simulink model "Motor_Position"  (R2020b)
settings: Solver=ode15s  StartTime=0.0  StopTime=0.2  RelTol=1e-3
undefined symbols (not defined in the file): b, J, Ke, Kt, L, R
settings Model: DataDictionary=motor_pos_data.sldd  Creator=ADMIN  LastModifiedBy=ADMIN
settings DataIOCC: SaveOutput=off  SaveTime=off

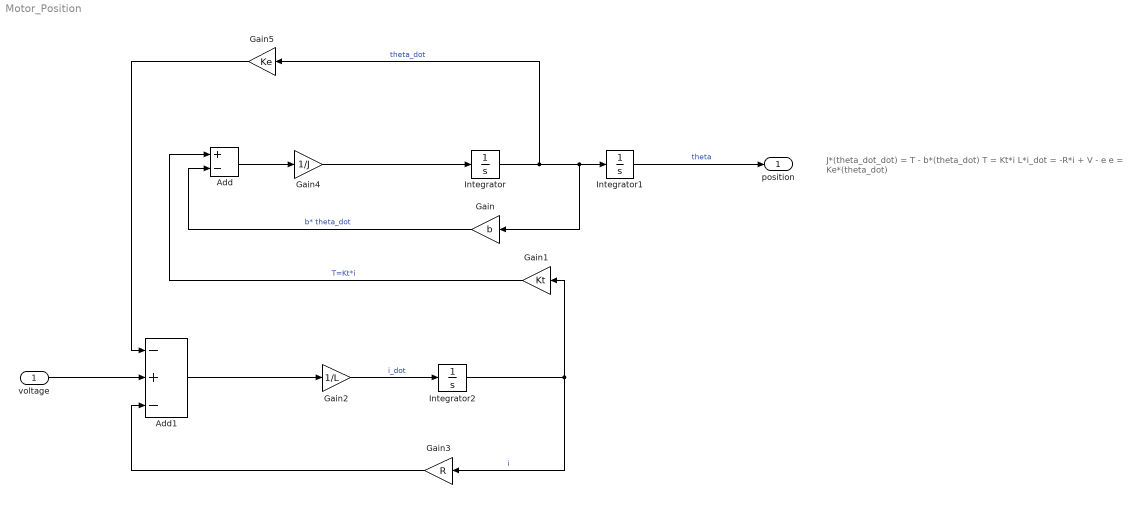
== system Motor_Position ==
  note: J*(theta_dot_dot) = T - b*(theta_dot)
      |
      | T = Kt*i
      |
      | L*i_dot = -R*i + V - e
      |
      | e = Ke*(theta_dot)
  voltage : Inport  OutDataTypeStr=double  PortDimensions=1
  Add : Sum  Inputs=+-
  Add1 : Sum  Inputs=-+-
  Gain : Gain  Gain=b
  Gain1 : Gain  Gain=Kt
  Gain2 : Gain  Gain=1/L
  Gain3 : Gain  Gain=R
  Gain4 : Gain  Gain=1/J
  Gain5 : Gain  Gain=Ke
  Integrator : Integrator
  Integrator1 : Integrator
  Integrator2 : Integrator
  position : Outport  OutDataTypeStr=double  PortDimensions=1  SampleTime=0
  wires:
  Add1/1 -> Gain2/1
  Gain3/1 -> Add1/3
  Integrator1/1 -> position/1  "theta"
  Gain/1 -> Add/2  "b* theta_dot"
  Gain4/1 -> Integrator/1
  Integrator2/1 -> Gain3/1, Gain1/1  "i"
  Integrator/1 -> Gain5/1, Integrator1/1, Gain/1  "theta_dot"
  Gain2/1 -> Integrator2/1  "i_dot"
  Gain5/1 -> Add1/1
  Gain1/1 -> Add/1  "T=Kt*i"
  voltage/1 -> Add1/2
  Add/1 -> Gain4/1
